simulink model "NoseHoover"  (R2014b)
settings: Solver=ode45  StartTime=0.0  StopTime=10.0  RelTol=1e-3
undefined symbols (not defined in the file or in its folder): param
settings Model: Creator=Arek  LastModifiedBy=Arek

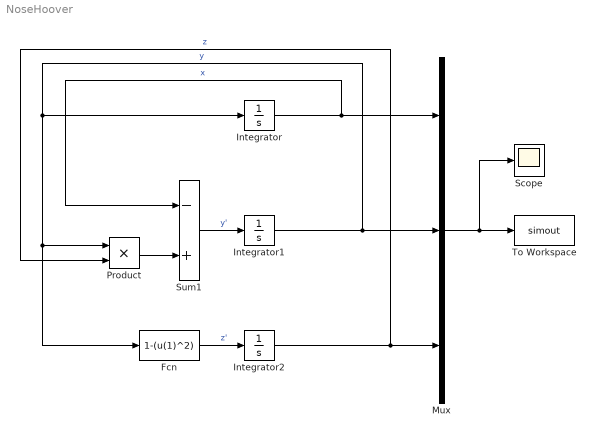
== system NoseHoover ==
  Fcn : Fcn  Expr=1-(u(1)^2)
  Integrator : Integrator  InitialCondition=param.ic(1)
  Integrator1 : Integrator  InitialCondition=param.ic(2)
  Integrator2 : Integrator  InitialCondition=param.ic(3)
  Mux : Mux  Inputs=3
  Product : Product
  Scope : Scope
      settings: ShowLegends=on
  Sum1 : Sum  Inputs=-+
  To Workspace : ToWorkspace  VariableName=simout  SaveFormat=Timeseries  SampleTime=-1
  wires:
  Integrator1/1 -> Mux/2, Integrator/1, Fcn/1, Product/1  "y"
  Integrator/1 -> Sum1/1, Mux/1  "x"
  Sum1/1 -> Integrator1/1  "y'"
  Fcn/1 -> Integrator2/1  "z'"
  Integrator2/1 -> Mux/3, Product/2  "z"
  Mux/1 -> To Workspace/1, Scope/1
  Product/1 -> Sum1/2
